simulink library "halin"  (R2021b)
settings: Solver=VariableStepAuto  StartTime=0.0  StopTime=10.0  RelTol=1e-3
undefined symbols (not defined in the file): TRUE
libraries: FVT_lib x100, hcu_lib x41
(part 10 of 10)

== system halin/HAL_IN/CAN5/TBOX2/TimeSyncFromBSDay ==
  TimeSyncFromBS_Day : Inport
  UnitConverter : DataTypeConversion  OutDataTypeStr=uint8
  VHAL_TimeSyncFromBSDay_DAY : Outport
  wires:
  UnitConverter/1 -> VHAL_TimeSyncFromBSDay_DAY/1
  TimeSyncFromBS_Day/1 -> UnitConverter/1

== system halin/HAL_IN/CAN5/TBOX2/TimeSyncFromBSHour ==
  TimeSyncFromBS_Hour : Inport
  UnitConverter : DataTypeConversion  OutDataTypeStr=uint8
  VHAL_TimeSyncFromBSHour_hr : Outport
  wires:
  UnitConverter/1 -> VHAL_TimeSyncFromBSHour_hr/1
  TimeSyncFromBS_Hour/1 -> UnitConverter/1

== system halin/HAL_IN/CAN5/TBOX2/TimeSyncFromBSMinute ==
  TimeSyncFromBS_Minute : Inport
  UnitConverter : DataTypeConversion  OutDataTypeStr=uint8
  VHAL_TimeSyncFromBSMinute_min : Outport
  wires:
  UnitConverter/1 -> VHAL_TimeSyncFromBSMinute_min/1
  TimeSyncFromBS_Minute/1 -> UnitConverter/1

== system halin/HAL_IN/CAN5/TBOX2/TimeSyncFromBSMonth ==
  TimeSyncFromBS_Month : Inport
  UnitConverter : DataTypeConversion  OutDataTypeStr=uint8
  VHAL_TimeSyncFromBSMonth_MONTH : Outport
  wires:
  UnitConverter/1 -> VHAL_TimeSyncFromBSMonth_MONTH/1
  TimeSyncFromBS_Month/1 -> UnitConverter/1

== system halin/HAL_IN/CAN5/TBOX2/TimeSyncFromBSSecond ==
  TimeSyncFromBS_Second : Inport
  UnitConverter : DataTypeConversion  OutDataTypeStr=uint8
  VHAL_TimeSyncFromBSSecond_s : Outport
  wires:
  UnitConverter/1 -> VHAL_TimeSyncFromBSSecond_s/1
  TimeSyncFromBS_Second/1 -> UnitConverter/1

== system halin/HAL_IN/CAN5/TBOX2/TimeSyncFromBSYear ==
  TimeSyncFromBS_Year : Inport
  UnitConverter : DataTypeConversion  OutDataTypeStr=uint8
  convert_in : FVT_lib/hal/convert_in  gain=1  offset=2000
  VHAL_TimeSyncFromBSYear_YEAR : Outport
  wires:
  convert_in/1 -> VHAL_TimeSyncFromBSYear_YEAR/1
  UnitConverter/1 -> convert_in/1
  TimeSyncFromBS_Year/1 -> UnitConverter/1

== system halin/HAL_IN/CAN5/TBOX3/ChargePercentSet ==
  Charge_Percent_Set : Inport
  UnitConverter : DataTypeConversion  OutDataTypeStr=uint8
  VHAL_ChargePercentSet_pct : Outport
  wires:
  UnitConverter/1 -> VHAL_ChargePercentSet_pct/1
  Charge_Percent_Set/1 -> UnitConverter/1

== system halin/HAL_IN/CAN5/TBOX3/ReserveChargeOFFDay ==
  ReserveChargeOFF_Day : Inport
  UnitConverter : DataTypeConversion  OutDataTypeStr=uint8
  VHAL_ReserveChargeOFFDay_DAY : Outport
  wires:
  UnitConverter/1 -> VHAL_ReserveChargeOFFDay_DAY/1
  ReserveChargeOFF_Day/1 -> UnitConverter/1

== system halin/HAL_IN/CAN5/TBOX3/ReserveChargeOFFHour ==
  ReserveChargeOFF_Hour : Inport
  UnitConverter : DataTypeConversion  OutDataTypeStr=uint8
  VHAL_ReserveChargeOFFHour_hr : Outport
  wires:
  UnitConverter/1 -> VHAL_ReserveChargeOFFHour_hr/1
  ReserveChargeOFF_Hour/1 -> UnitConverter/1

== system halin/HAL_IN/CAN5/TBOX3/ReserveChargeOFFMinute ==
  ReserveChargeOFF_Minute : Inport
  UnitConverter : DataTypeConversion  OutDataTypeStr=uint8
  VHAL_ReserveChargeOFFMinute_min : Outport
  wires:
  UnitConverter/1 -> VHAL_ReserveChargeOFFMinute_min/1
  ReserveChargeOFF_Minute/1 -> UnitConverter/1

== system halin/HAL_IN/CAN5/TBOX3/ReserveChargeOFFMonth ==
  ReserveChargeOFF_Month : Inport
  UnitConverter : DataTypeConversion  OutDataTypeStr=uint8
  VHAL_ReserveChargeOFFMonth_MONTH : Outport
  wires:
  UnitConverter/1 -> VHAL_ReserveChargeOFFMonth_MONTH/1
  ReserveChargeOFF_Month/1 -> UnitConverter/1

== system halin/HAL_IN/CAN5/TBOX3/ReserveChargeOFFYear ==
  ReserveChargeOFF_Year : Inport
  UnitConverter : DataTypeConversion  OutDataTypeStr=uint8
  convert_in : FVT_lib/hal/convert_in  gain=1  offset=2000
  VHAL_ReserveChargeOFFYear_YEAR : Outport
  wires:
  convert_in/1 -> VHAL_ReserveChargeOFFYear_YEAR/1
  UnitConverter/1 -> convert_in/1
  ReserveChargeOFF_Year/1 -> UnitConverter/1

== system halin/HAL_IN/CAN5/TBOX3/ReserveChargeOnDay ==
  ReserveChargeOn_Day : Inport
  UnitConverter : DataTypeConversion  OutDataTypeStr=uint8
  VHAL_ReserveChargeOnDay_DAY : Outport
  wires:
  UnitConverter/1 -> VHAL_ReserveChargeOnDay_DAY/1
  ReserveChargeOn_Day/1 -> UnitConverter/1

== system halin/HAL_IN/CAN5/TBOX3/ReserveChargeOnHour ==
  ReserveChargeOn_Hour : Inport
  UnitConverter : DataTypeConversion  OutDataTypeStr=uint8
  VHAL_ReserveChargeOnHour_hr : Outport
  wires:
  UnitConverter/1 -> VHAL_ReserveChargeOnHour_hr/1
  ReserveChargeOn_Hour/1 -> UnitConverter/1

== system halin/HAL_IN/CAN5/TBOX3/ReserveChargeOnMinute ==
  ReserveChargeOn_Minute : Inport
  UnitConverter : DataTypeConversion  OutDataTypeStr=uint8
  VHAL_ReserveChargeOnMinute_min : Outport
  wires:
  UnitConverter/1 -> VHAL_ReserveChargeOnMinute_min/1
  ReserveChargeOn_Minute/1 -> UnitConverter/1

== system halin/HAL_IN/CAN5/TBOX3/ReserveChargeOnMonth ==
  ReserveChargeOn_Month : Inport
  UnitConverter : DataTypeConversion  OutDataTypeStr=uint8
  VHAL_ReserveChargeOnMonth_MONTH : Outport
  wires:
  UnitConverter/1 -> VHAL_ReserveChargeOnMonth_MONTH/1
  ReserveChargeOn_Month/1 -> UnitConverter/1

== system halin/HAL_IN/CAN5/TBOX3/ReserveChargeOnYear ==
  ReserveChargeOn_Year : Inport
  UnitConverter : DataTypeConversion  OutDataTypeStr=uint8
  convert_in : FVT_lib/hal/convert_in  gain=1  offset=2000
  VHAL_ReserveChargeOnYear_YEAR : Outport
  wires:
  convert_in/1 -> VHAL_ReserveChargeOnYear_YEAR/1
  UnitConverter/1 -> convert_in/1
  ReserveChargeOn_Year/1 -> UnitConverter/1

== system halin/HAL_IN/CAN5/TBOX3/TBOXHWVER ==
  TBOX_HW_VER : Inport
  UnitConverter : DataTypeConversion  OutDataTypeStr=uint32
  VHAL_TBOXHWVER_enum : Outport
  wires:
  UnitConverter/1 -> VHAL_TBOXHWVER_enum/1
  TBOX_HW_VER/1 -> UnitConverter/1

== system halin/HAL_IN/CAN5/TBOX3/TBOXSWVER ==
  TBOX_SW_VER : Inport
  UnitConverter : DataTypeConversion  OutDataTypeStr=uint32
  VHAL_TBOXSWVER_enum : Outport
  wires:
  UnitConverter/1 -> VHAL_TBOXSWVER_enum/1
  TBOX_SW_VER/1 -> UnitConverter/1

== system halin/HAL_IN/CAN7/Door_Fr1/DoorFrDoorEmergencysta ==
  Door_Fr_DoorEmergency_sta : Inport
  UnitConverter : DataTypeConversion  OutDataTypeStr=uint8
  VHAL_DoorFrDoorEmergencysta_enum : Outport
  wires:
  UnitConverter/1 -> VHAL_DoorFrDoorEmergencysta_enum/1
  Door_Fr_DoorEmergency_sta/1 -> UnitConverter/1

== system halin/HAL_IN/CAN7/Door_Fr1/DoorFrDooroperationsta ==
  Door_Fr_Dooroperation_sta : Inport
  UnitConverter : DataTypeConversion  OutDataTypeStr=uint8
  VHAL_DoorFrDooroperationsta_enum : Outport
  wires:
  UnitConverter/1 -> VHAL_DoorFrDooroperationsta_enum/1
  Door_Fr_Dooroperation_sta/1 -> UnitConverter/1

== system halin/HAL_IN/CAN7/Door_Fr1/DoorFrDoorpositionsta ==
  Door_Fr_Doorposition_sta : Inport
  UnitConverter : DataTypeConversion  OutDataTypeStr=uint8
  VHAL_DoorFrDoorpositionsta_enum : Outport
  wires:
  UnitConverter/1 -> VHAL_DoorFrDoorpositionsta_enum/1
  Door_Fr_Doorposition_sta/1 -> UnitConverter/1
